simulink model "HVDC_system_original"  (R2024b)
settings: Solver=FixedStepDiscrete  StartTime=0.0  StopTime=1.5  RelTol=1e-4  EnableMultiTasking=on
PreLoadFcn:
  | power_converters_init;
values from neighbouring files (symbols this model uses):
  Clink_3L = Pnom_dc_3L*H_3L*2 /Vnom_dc_3L^2    (= 0.0111111111111)    [HVDC_system_init_original.m]
  fault_distance_km = fault.dist_km    [HVDC_system_init_original.m]
  Fnom = 60    [HVDC_system_init_original.m]
  Ki_Ireg_3L = 15    [HVDC_system_init_original.m]
  Ki_VDCreg_3L = 300    [HVDC_system_init_original.m]
  Kp_Ireg_3L = 0.2/2    (= 0.1)    [HVDC_system_init_original.m]
  Kp_VDCreg_3L = 3    [HVDC_system_init_original.m]
  LimitL_Ireg_3L = -1.5    [HVDC_system_init_original.m]
  LimitL_VDCreg_3L = -1.5    [HVDC_system_init_original.m]
  LimitU_Ireg_3L = 1.5    [HVDC_system_init_original.m]
  LimitU_VDCreg_3L = 1.5    [HVDC_system_init_original.m]
  Lxfo_3L = 0.10    (= 0.1)    [HVDC_system_init_original.m]
  n_g_switch_time = NEVER_TIME    (= 999)    [HVDC_system_init_original.m]
  p_g_switch_time = NEVER_TIME    (= 999)    [HVDC_system_init_original.m]
  p_n_switch_time = NEVER_TIME    (= 999)    [HVDC_system_init_original.m]
  Pnom_3L = Pnom_dc_3L    (= 3000000)    [HVDC_system_init_original.m]
  Pnom_dc_3L = 3e6    (= 3000000)    [HVDC_system_init_original.m]
  Psc_grid = 200e6    (= 200000000)    [HVDC_system_init_original.m]
  R_fault = fault.R    [HVDC_system_init_original.m]
  Rxfo_3L = 0.10/30    (= 0.00333333333333)    [HVDC_system_init_original.m]
  Ts_Control = 50e-6    (= 5e-05)    [HVDC_system_init_original.m]
  Ts_Power = Ts_PWM    (= 5e-06)    [HVDC_system_init_original.m]
  Ts_PWM = 5e-6    (= 5e-06)    [HVDC_system_init_original.m]
  Vnom_dc_3L = 3000    [HVDC_system_init_original.m]
  Vnom_grid = 50e3    (= 50000)    [HVDC_system_init_original.m]
  Vnom_prim_3L = Vnom_grid    (= 50000)    [HVDC_system_init_original.m]
  Vnom_sec_3L = 0.5*Vnom_dc_3L/sqrt(2)*sqrt(3)*m_nom_3L    [HVDC_system_init_original.m]
undefined symbols (not defined in the file or in its folder): D1, Delta, DiscIntNeverNeededParam
libraries: spsSeriesRLCBranchLib x11, powerlib_extras x9, spsVoltageMeasurementLib x8, spsGroundLib x6, spsBreakerLib x4, spsabctodq0Lib x4, spsMeanLib x4, spsPiSectionLineLib x4, spsSecondOrderFilterLib x3, spsThreePhaseVIMeasurementLib x3, spsPLL3phLib x2, spsPWMGenerator3LevelLib x2
(part 1 of 2)
Description:
  | Copyright 2008-2015 The MathWorks, Inc.
settings Model: Creator=MathWorks  LastModifiedBy=ccart030
settings SolverCC: AlgebraicLoopSolver=TrustRegion  AutoInsertRateTranBlk=on
settings DataIOCC: SaveFormat=Array  SaveOutput=off  SignalLogging=off  DSMLogging=off  SaveTime=off  ReturnWorkspaceOutputs=off
settings OptimizationCC: ExpressionDepthLimit=2147483647  LifeSpan=inf
settings DebuggingCC: ConsistencyChecking=warning  UnderspecifiedInitializationDetection=Classic  MergeDetectMultiDrivingBlocksExec=none  TimeAdjustmentMsg=warning  SingleTaskRateTransMsg=warning  VectorMatrixConversionMsg=warning  UnconnectedInputMsg=warning  UnconnectedOutputMsg=warning  UnconnectedLineMsg=warning  AllowSymbolicDim=off  ModelReferenceIOMismatchMessage=warning  StateNameClashWarn=warning  StrictBusMsg=WarnOnBusTreatedAsVector  NonBusSignalsTreatedAsBus=warning  SFUnexpectedBacktrackingDiag=warning  SFNoUnconditionalDefaultTransitionDiag=warning  SFExecutionAtInitializationDiag=none  ArithmeticOperatorsInVariantConditions=warning
settings HardwareCC: ProdBitPerPointer=32  ProdBitPerSizeT=32  ProdBitPerPtrDiffT=32  ProdLargestAtomicFloat=None  ProdIntDivRoundTo=Undefined  ProdEndianess=Unspecified  ProdWordSize=32  ProdHWDeviceType=32-bit Generic
settings ModelReferenceCC: EnableRefExpFcnMdlSchedulingChecks=on  PropagateSignalLabelsOutOfModel=off
settings SFSimCC: SimUseLocalCustomCode=off  CustomCodeUndefinedFunction=UseInterfaceOnly
settings RTWCC: RTWUseLocalCustomCode=off  GPUComputeCapability=3.5
settings CodeAppCC: StateflowObjectComments=on
settings GRTTargetCC: TargetLangStandard=C89/C90 (ANSI)
settings ConfigComp: CovMetricSettings=dw  CovSaveCumulativeToWorkspaceVar=on  CovSaveSingleToWorkspaceVar=on  CovExternalEMLEnable=off  CovSFcnEnable=off
settings SimscapeCC: SimscapeNormalizeSystem=off

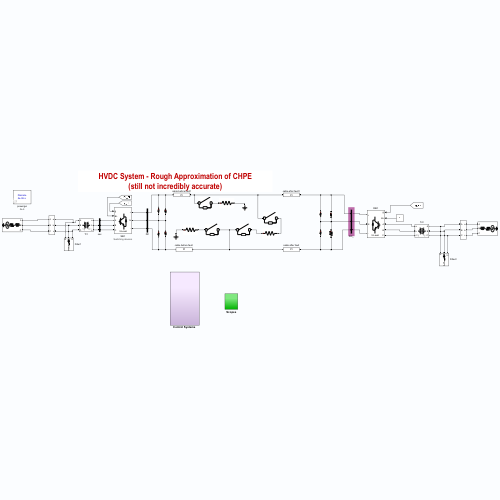
[thumbnail: Simulink's stored preview of the top-level diagram]
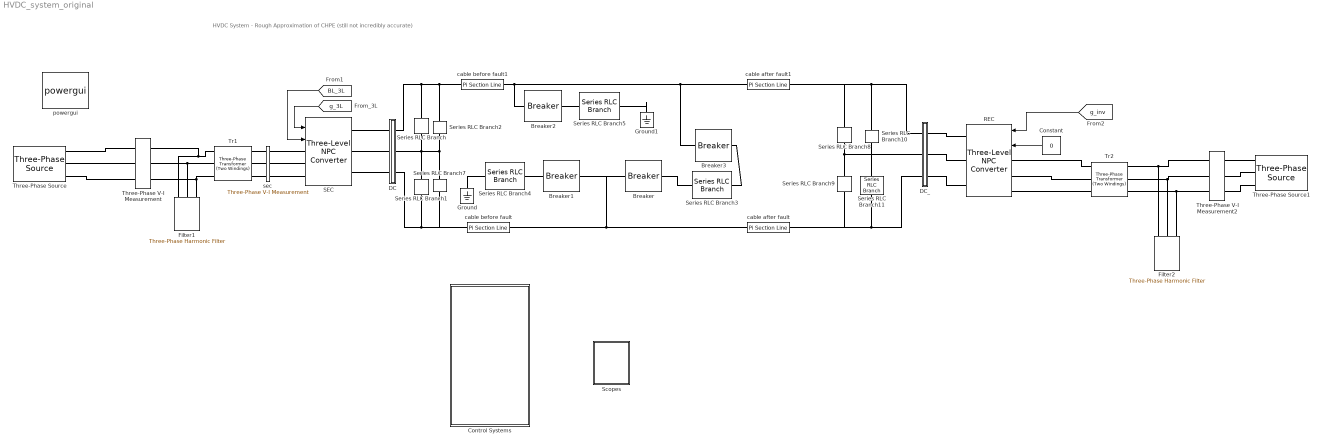
== system HVDC_system_original ==
  note: HVDC System - Rough Approximation of CHPE
      | (still not incredibly accurate)
  Breaker : spsBreakerLib/Breaker  InitialState=0  SwitchingTimes=[p_n_switch_time]  External=off  BreakerResistance=0.01  SnubberResistance=1e6  SnubberCapacitance=inf  Measurements=None  MoreParameters=on  NoBreakLoop=off
  Breaker1 : spsBreakerLib/Breaker  InitialState=0  SwitchingTimes=[n_g_switch_time]  External=off  BreakerResistance=0.01  SnubberResistance=1e6  SnubberCapacitance=inf  Measurements=None  MoreParameters=on  NoBreakLoop=off
  Breaker2 : spsBreakerLib/Breaker  InitialState=0  SwitchingTimes=[p_g_switch_time]  External=off  BreakerResistance=0.01  SnubberResistance=1e6  SnubberCapacitance=inf  Measurements=None  MoreParameters=on  NoBreakLoop=off
  Breaker3 : spsBreakerLib/Breaker  InitialState=0  SwitchingTimes=[p_n_switch_time]  External=off  BreakerResistance=0.01  SnubberResistance=1e6  SnubberCapacitance=inf  Measurements=None  MoreParameters=on  NoBreakLoop=off
  Constant : Constant  Value=0
  "Control Systems " : Subsystem
  DC : Subsystem
  DC_ : Subsystem
  Filter1 : spsThreePhaseHarmonicFilterLib/Three-Phase Harmonic Filter  LConnTagsString=A|B|C  FilterType=Single-tuned  FilterConnection=Y (grounded)  ParNom=[Vnom_prim_3L Fnom]  Qc=Qnom_Filter1  Fr=Fn_Filter1  Frd=[11*60 13*60]  Q=Q_Filter1  Measurements=None
      settings: AttributesFormatString=\n
      settings: LibrarySourceBlock=|
      | sps_lib/Passives/Three-Phase
      | Harmonic Filter
  Filter2 : spsThreePhaseHarmonicFilterLib/Three-Phase Harmonic Filter  LConnTagsString=A|B|C  FilterType=Single-tuned  FilterConnection=Y (grounded)  ParNom=[Vnom_prim_3L Fnom]  Qc=Qnom_Filter1  Fr=Fn_Filter1  Frd=[11*60 13*60]  Q=Q_Filter1  Measurements=None
      settings: AttributesFormatString=\n
      settings: LibrarySourceBlock=|
      | sps_lib/Passives/Three-Phase
      | Harmonic Filter
  Ground : spsGroundLib/Ground  LConnTagsString=a
  Ground1 : spsGroundLib/Ground  LConnTagsString=a
  REC : spsThreeLevelNPCConverterLib/Three-Level NPC Converter  ModelType=Switching devices  Ron=1e-3  Rs=1e6  Cs=inf  Vforward=[0,0]  Ron_Diode=1e-3  Rs_Diode=1e6  Cs_Diode=inf  Vf_Diode=1e-3  Rs_CurrentSource=inf  Ron_ACsource=1e-3
      settings: LibrarySourceBlock=|
      | sps_lib/Power Electronics/Three-Level
      | NPC Converter
  SEC : spsThreeLevelNPCConverterLib/Three-Level NPC Converter  ModelType=Switching devices  Ron=1e-3  Rs=1e6  Cs=inf  Vforward=[ 0, 0 ]  Ron_Diode=1e-3  Rs_Diode=1e6  Cs_Diode=inf  Vf_Diode=1e-3  Rs_CurrentSource=inf  Ron_ACsource=1e-3
      settings: AttributesFormatString=%<ModelType>
      settings: LibrarySourceBlock=|
      | sps_lib/Power Electronics/Three-Level
      | NPC Converter
  Scopes : Subsystem
  Series RLC Branch : spsSeriesRLCBranchLib/Series RLC Branch  LConnTagsString=__new0  RConnTagsString=__new0  BranchType=C  Resistance=1  Inductance=1e-3  SetiL0=off  InitialCurrent=0  Capacitance=Clink_3L  Setx0=on  InitialVoltage=Vc_Initial_3L  Measurements=None
  Series RLC Branch1 : spsSeriesRLCBranchLib/Series RLC Branch  LConnTagsString=__new0  RConnTagsString=__new0  BranchType=C  Resistance=1  Inductance=1e-3  SetiL0=off  InitialCurrent=0  Capacitance=Clink_3L  Setx0=on  InitialVoltage=Vc_Initial_3L  Measurements=None
  Series RLC Branch{2,7,10..11} (4 alike) : spsSeriesRLCBranchLib/Series RLC Branch  LConnTagsString=__new0  RConnTagsString=__new0  BranchType=R  Resistance=Vnom_dc_3L^2/(Pnom_dc_3L*0.01)/2  Inductance=1e-3  SetiL0=off  InitialCurrent=0  Capacitance=1e-6  Setx0=off  InitialVoltage=0  Measurements=None
  Series RLC Branch3 : spsSeriesRLCBranchLib/Series RLC Branch  LConnTagsString=__new0  RConnTagsString=__new0  BranchType=R  Resistance=R_fault  Inductance=1e-3  SetiL0=off  InitialCurrent=0  Capacitance=1e-6  Setx0=off  InitialVoltage=0  Measurements=None
  Series RLC Branch4 : spsSeriesRLCBranchLib/Series RLC Branch  LConnTagsString=__new0  RConnTagsString=__new0  BranchType=R  Resistance=R_fault  Inductance=1e-3  SetiL0=off  InitialCurrent=0  Capacitance=1e-6  Setx0=off  InitialVoltage=0  Measurements=None
  Series RLC Branch5 : spsSeriesRLCBranchLib/Series RLC Branch  LConnTagsString=__new0  RConnTagsString=__new0  BranchType=R  Resistance=R_fault  Inductance=1e-3  SetiL0=off  InitialCurrent=0  Capacitance=1e-6  Setx0=off  InitialVoltage=0  Measurements=None
  Series RLC Branch8 : spsSeriesRLCBranchLib/Series RLC Branch  LConnTagsString=__new0  RConnTagsString=__new0  BranchType=C  Resistance=1  Inductance=1e-3  SetiL0=off  InitialCurrent=0  Capacitance=Clink_3L  Setx0=on  InitialVoltage=Vc_Initial_3L  Measurements=None
  Series RLC Branch9 : spsSeriesRLCBranchLib/Series RLC Branch  LConnTagsString=__new0  RConnTagsString=__new0  BranchType=C  Resistance=1  Inductance=1e-3  SetiL0=off  InitialCurrent=0  Capacitance=Clink_3L  Setx0=off  InitialVoltage=1000  Measurements=None
  Three-Phase V-I Measurement : spsThreePhaseVIMeasurementLib/Three-Phase V-I Measurement  VoltageMeasurement=phase-to-ground  SetLabelV=on  LabelV=Vgrid  Vpu=off  VpuLL=off  CurrentMeasurement=yes  SetLabelI=on  LabelI=Igrid  Ipu=off  Pbase=100e6  Vbase=500e3  OutputType=Complex  PhasorSimulation=off  PSBequivalent=0
  Three-Phase V-I Measurement2 : spsThreePhaseVIMeasurementLib/Three-Phase V-I Measurement  VoltageMeasurement=phase-to-ground  SetLabelV=on  LabelV=Uinv  Vpu=off  VpuLL=off  CurrentMeasurement=yes  SetLabelI=on  LabelI=Iinv  Ipu=off  Pbase=100e6  Vbase=500e3  OutputType=Complex  PhasorSimulation=off  PSBequivalent=0
  Three-Phase Source : spsThreePhaseSourceLib/Three-Phase Source  InternalConnection=Yg  VoltagePhases=off  Voltage=Vnom_grid  PhaseAngle=0  Voltage_phases=[25e3 25e3 25e3]/sqrt(3)  PhaseAngles_phases=[0 -120 +120]  Frequency=Fnom  NonIdealSource=on  SpecifyImpedance=off  Resistance=Vnom_grid*Vnom_grid/Psc_grid/7  Inductance=Vnom_grid*Vnom_grid/Psc_grid/(2*pi*Fnom)  ShortCircuitLevel=100e6  BaseVoltage=Vnom_grid  XRratio=7  BusType=swing  Pref=10e3  Qref=0  Prefabc=[10e3, 10e3, 10e3]  Qrefabc=[0, 0, 0]  Qmin=-inf  Qmax=inf
  Three-Phase Source1 : spsThreePhaseSourceLib/Three-Phase Source  InternalConnection=Yg  VoltagePhases=off  Voltage=Vnom_grid  PhaseAngle=0  Voltage_phases=[25e3 25e3 25e3]/sqrt(3)  PhaseAngles_phases=[0 -120 +120]  Frequency=Fnom  NonIdealSource=on  SpecifyImpedance=off  Resistance=Vnom_grid*Vnom_grid/Psc_grid/7  Inductance=Vnom_grid*Vnom_grid/Psc_grid/(2*pi*Fnom)  ShortCircuitLevel=100e6  BaseVoltage=Vnom_grid  XRratio=7  BusType=swing  Pref=10e3  Qref=0  Prefabc=[10e3, 10e3, 10e3]  Qrefabc=[0, 0, 0]  Qmin=-inf  Qmax=inf
  Tr1 : spsThreePhaseTransformerTwoWindingsLib/Three-Phase Transformer (Two Windings)  Winding1Connection=Yg  Winding2Connection=Delta (D1)  CoreType=Three single-phase transformers  SetSaturation=off  Hysteresis=off  DataFile='hysteresis'  SetInitialFlux=off  Measurements=None  UNITS=pu  NominalPower="[ Pnom_3L,  Fnom ]"  Winding1=[ Vnom_prim_3L ,Rxfo_3L/2 Lxfo_3L/2 ]  Winding2=[ Vnom_sec_3L ,Rxfo_3L/2 Lxfo_3L/2 ]  Rm=Rm_3L  Lm=Lm_3L  L0=0.5  Saturation=[ 0,0 ; 0.0024,1.2 ; 1.0,1.52 ]  InitialFluxes=[ 0.8 , -0.8 , 0.7 ]  BreakLoop=off  DiscreteSolver=Trapezoidal iterative  DataType=off  TransfoNumber=1
  Tr2 : spsThreePhaseTransformerTwoWindingsLib/Three-Phase Transformer (Two Windings)  Winding1Connection=Yg  Winding2Connection=Yg  CoreType=Three single-phase transformers  SetSaturation=off  Hysteresis=off  DataFile='hysteresis'  SetInitialFlux=off  Measurements=None  UNITS=pu  NominalPower="[ Pnom_3L,  Fnom ]"  Winding1=[ Vnom_prim_3L ,Rxfo_3L/2 Lxfo_3L/2 ]  Winding2=[ Vnom_sec_3L ,Rxfo_3L/2 Lxfo_3L/2 ]  Rm=Rm_3L  Lm=Lm_3L  L0=0.5  Saturation=[ 0,0 ; 0.0024,1.2 ; 1.0,1.52 ]  InitialFluxes=[ 0.8 , -0.8 , 0.7 ]  BreakLoop=off  DiscreteSolver=Trapezoidal iterative  DataType=off  TransfoNumber=1
  cable after fault : spsPiSectionLineLib/Pi Section Line  LConnTagsString=__new0  RConnTagsString=__new0  Phases=1  PiSections=2  Length=546-fault_distance_km  Frequency=Fnom  Resistance=1.3900e-004  Inductance=1.5900e-005  Capacitance=2.3100e-005  SpecifyConductance=off  Conductance=0  Measurements=None  Measurements2=None
      settings: LibrarySourceBlock=sps_lib/Power Grid Elements/Pi Section Line
  cable after fault1 : spsPiSectionLineLib/Pi Section Line  LConnTagsString=__new0  RConnTagsString=__new0  Phases=1  PiSections=2  Length=546-fault_distance_km  Frequency=Fnom  Resistance=1.3900e-004  Inductance=1.5900e-005  Capacitance=2.3100e-005  SpecifyConductance=off  Conductance=0  Measurements=None  Measurements2=None
      settings: LibrarySourceBlock=sps_lib/Power Grid Elements/Pi Section Line
  "cable before fault " : spsPiSectionLineLib/Pi Section Line  LConnTagsString=__new0  RConnTagsString=__new0  Phases=1  PiSections=2  Length=fault_distance_km  Frequency=Fnom  Resistance=1.3900e-004  Inductance=1.5900e-005  Capacitance=2.3100e-005  SpecifyConductance=off  Conductance=0  Measurements=None  Measurements2=None
      settings: LibrarySourceBlock=sps_lib/Power Grid Elements/Pi Section Line
  cable before fault1 : spsPiSectionLineLib/Pi Section Line  LConnTagsString=__new0  RConnTagsString=__new0  Phases=1  PiSections=2  Length=fault_distance_km  Frequency=Fnom  Resistance=1.3900e-004  Inductance=1.5900e-005  Capacitance=2.3100e-005  SpecifyConductance=off  Conductance=0  Measurements=None  Measurements2=None
      settings: LibrarySourceBlock=sps_lib/Power Grid Elements/Pi Section Line
  powergui : sps_lib/powergui  Priority=1  SimulationMode=Discrete  SampleTime=5e-6  frequency=60  Iterations=50  frequencyindice=60  Pbase=100e6  ErrMax=1e-4  UnitsV=kV  UnitsW=MW  buscounter=0  FunctionMessages=off  echomessages=off  EnableUseOfTLC=off  CurrentSourceSwitches=off  DisableSnubberDevices=off  DisableRonSwitches=off  DisableVfSwitches=off  DisplayEquations=off  AutomaticDiscreteSolvers=off  SolverType=Tustin/Backward Euler (TBE)  Interpol=off  ExternalGateDelay=off  methode=on  Ts=100  x0status=steady  SPID=off  SwTol=0  HookPort=off  NonlinearTolerance=1e-4  nMaxIteration=100  ContinueOnMaxIteration=off  RestoreLinks=warning  ResistiveCurrentMeasurement=off  Frange=[0:2:500]  Ylog=off  Xlog=on  ShowGrid=off  save=off  variable=ZData  structure=VIPFB  ZoomFFT=on  StartTime=0.87  cycles=1  DisplayStyle=1  fundamental=50  FreqAxis=on  MaxFrequency=5000  frequencyindicesteady=1  RmsSteady=2  display=off
      settings: AttributesFormatString=%<SampleTime>
  sec : spsThreePhaseVIMeasurementLib/Three-Phase V-I Measurement  VoltageMeasurement=phase-to-phase  SetLabelV=on  LabelV=Vsec_3L_LL  Vpu=off  VpuLL=off  CurrentMeasurement=no  SetLabelI=on  LabelI=Isec  Ipu=off  Pbase=100e6  Vbase=500e3  OutputType=Complex  PhasorSimulation=off  PSBequivalent=0
  wires:
  [g_3L] -> SEC/1
  [BL_3L] -> SEC/2
  Constant/1 -> REC/2
  [g_inv] -> REC/1
  connections:
  Filter1/LConn1 -- Three-Phase V-I Measurement/RConn1 -- Tr1/LConn1
  Filter1/LConn3 -- Three-Phase V-I Measurement/RConn3 -- Tr1/LConn3
  sec/RConn1 -- Tr1/RConn1
  Tr1/RConn2 -- sec/RConn2
  Tr1/RConn3 -- sec/RConn3
  SEC/LConn1 -- sec/LConn1
  SEC/LConn2 -- sec/LConn2
  SEC/LConn3 -- sec/LConn3
  Three-Phase Source/RConn1 -- Three-Phase V-I Measurement/LConn1
  Three-Phase Source/RConn2 -- Three-Phase V-I Measurement/LConn2
  Three-Phase Source/RConn3 -- Three-Phase V-I Measurement/LConn3
  SEC/RConn1 -- DC/LConn1
  SEC/RConn2 -- DC/LConn2
  SEC/RConn3 -- DC/LConn3
  Series RLC Branch1/RConn1 -- Series RLC Branch7/RConn1 -- "cable before fault "/LConn1 -- DC/RConn3
  Series RLC Branch1/LConn1 -- DC/RConn2 -- Series RLC Branch7/LConn1 -- Series RLC Branch2/RConn1 -- Series RLC Branch/RConn1
  Filter1/LConn2 -- Three-Phase V-I Measurement/RConn2 -- Tr1/LConn2
  Tr2/RConn1 -- REC/LConn1
  REC/LConn2 -- Tr2/RConn2
  REC/LConn3 -- Tr2/RConn3
  DC_/RConn1 -- REC/RConn1
  DC_/RConn2 -- REC/RConn2
  DC_/RConn3 -- REC/RConn3
  Series RLC Branch8/RConn1 -- Series RLC Branch11/LConn1 -- DC_/LConn2 -- Series RLC Branch10/RConn1 -- Series RLC Branch9/LConn1
  Series RLC Branch2/LConn1 -- cable before fault1/LConn1 -- DC/RConn1 -- Series RLC Branch/LConn1
  Three-Phase V-I Measurement2/LConn2 -- Filter2/LConn2 -- Tr2/LConn2
  Three-Phase V-I Measurement2/LConn1 -- Tr2/LConn1 -- Filter2/LConn1
  Three-Phase V-I Measurement2/LConn3 -- Filter2/LConn3 -- Tr2/LConn3
  Three-Phase Source1/RConn1 -- Three-Phase V-I Measurement2/RConn1
  Three-Phase Source1/RConn2 -- Three-Phase V-I Measurement2/RConn2
  Three-Phase Source1/RConn3 -- Three-Phase V-I Measurement2/RConn3
  Series RLC Branch10/LConn1 -- cable after fault1/RConn1 -- Series RLC Branch8/LConn1 -- DC_/LConn1
  Series RLC Branch11/RConn1 -- Series RLC Branch9/RConn1 -- cable after fault/RConn1 -- DC_/LConn3
  "cable before fault "/RConn1 -- Breaker/LConn1 -- Breaker1/RConn1 -- cable after fault/LConn1
  cable before fault1/RConn1 -- Breaker3/LConn1 -- cable after fault1/LConn1 -- Breaker2/LConn1
  Breaker/RConn1 -- Series RLC Branch3/LConn1
  Series RLC Branch4/RConn1 -- Breaker1/LConn1
  Series RLC Branch3/RConn1 -- Breaker3/RConn1
  Ground/LConn1 -- Series RLC Branch4/LConn1
  Series RLC Branch5/LConn1 -- Breaker2/RConn1
  Ground1/LConn1 -- Series RLC Branch5/RConn1

== system HVDC_system_original/Control Systems  ==
  REC Control : Subsystem
  SEC Control : Subsystem

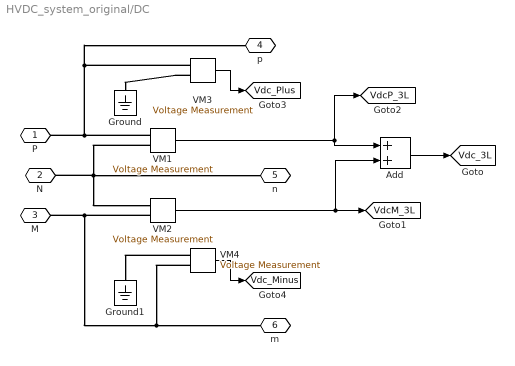
== system HVDC_system_original/DC ==
  Add : Sum
  Ground : spsGroundLib/Ground  LConnTagsString=a
  Ground1 : spsGroundLib/Ground  LConnTagsString=a
  VM{1..4} (4 alike) : spsVoltageMeasurementLib/Voltage Measurement  PhasorSimulation=off  OutputType=Complex  PSBequivalent=0
  P : PMIOPort  Side=Left
  N : PMIOPort  Port=2  Side=Left
  M : PMIOPort  Port=3  Side=Left
  p : PMIOPort  Port=4  Side=Right
  n : PMIOPort  Port=5  Side=Right
  m : PMIOPort  Port=6  Side=Right
  tag scope: VdcM_3L=global, VdcP_3L=global, Vdc_3L=global, Vdc_Minus=global, Vdc_Plus=global
  wires:
  VM1/1 -> [VdcP_3L], Add/1
  VM2/1 -> Add/2, [VdcM_3L]
  Add/1 -> [Vdc_3L]
  VM3/1 -> [Vdc_Plus]
  VM4/1 -> [Vdc_Minus]
  connections:
  VM1/LConn1 -- VM3/LConn1 -- p/RConn1 -- P/RConn1
  VM2/LConn2 -- VM4/LConn2 -- m/RConn1 -- M/RConn1
  VM1/LConn2 -- n/RConn1 -- VM2/LConn1 -- N/RConn1
  VM3/LConn2 -- Ground/LConn1
  VM4/LConn1 -- Ground1/LConn1

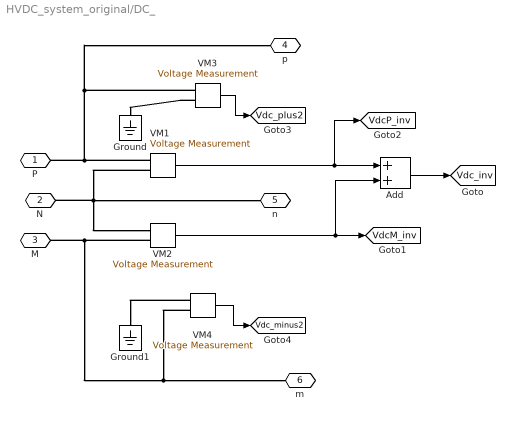
== system HVDC_system_original/DC_ ==
  Add : Sum
  Ground : spsGroundLib/Ground  LConnTagsString=a
  Ground1 : spsGroundLib/Ground  LConnTagsString=a
  VM{1..4} (4 alike) : spsVoltageMeasurementLib/Voltage Measurement  PhasorSimulation=off  OutputType=Complex  PSBequivalent=0
  P : PMIOPort  Side=Left
  N : PMIOPort  Port=2  Side=Left
  M : PMIOPort  Port=3  Side=Left
  p : PMIOPort  Port=4  Side=Right
  n : PMIOPort  Port=5  Side=Right
  m : PMIOPort  Port=6  Side=Right
  tag scope: VdcM_inv=global, VdcP_inv=global, Vdc_inv=global, Vdc_minus2=global, Vdc_plus2=global
  wires:
  VM1/1 -> [VdcP_inv], Add/1
  VM2/1 -> Add/2, [VdcM_inv]
  Add/1 -> [Vdc_inv]
  VM3/1 -> [Vdc_plus2]
  VM4/1 -> [Vdc_minus2]
  connections:
  VM1/LConn1 -- VM3/LConn1 -- p/RConn1 -- P/RConn1
  VM2/LConn2 -- VM4/LConn2 -- m/RConn1 -- M/RConn1
  VM1/LConn2 -- n/RConn1 -- VM2/LConn1 -- N/RConn1
  VM3/LConn2 -- Ground/LConn1
  VM4/LConn1 -- Ground1/LConn1

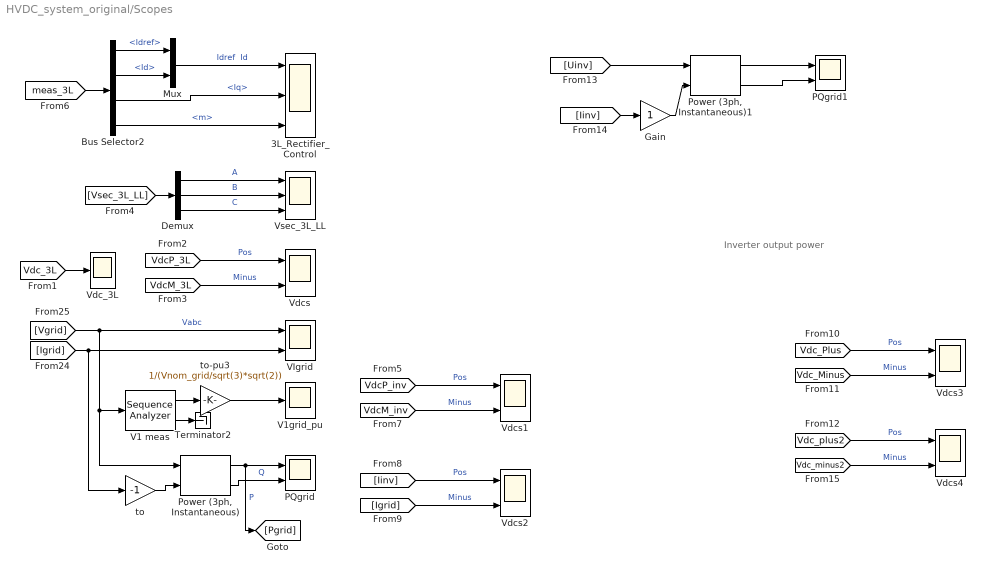
== system HVDC_system_original/Scopes ==
  note: Inverter output power
  3L_Rectifier_Control : Scope  NumInputPorts=3
  Bus Selector2 : BusSelector  OutputSignals=Idref,Id,Iq,m
  Demux : Demux  Outputs=3
  Gain : Gain
  Mux : Mux  Inputs=2
  PQgrid : Scope  NumInputPorts=2
  PQgrid1 : Scope  NumInputPorts=2
  "Power (3ph, Instantaneous)" : spsPower3phInstantaneousLib/Power (3ph, Instantaneous)
  "Power (3ph, Instantaneous)1" : spsPower3phInstantaneousLib/Power (3ph, Instantaneous)
  Terminator2 : Terminator
  V1 meas : spsSequenceAnalyzerLib/Sequence Analyzer  Freq=Fnom  n=1  seq=Positive  InInit=[1, 0]  Ts=Ts_Power
      settings: LibrarySourceBlock=sps_lib/Sensors and Measurements/Sequence Analyzer
  V1grid_pu : Scope
  VIgrid : Scope  NumInputPorts=2
  Vdc_3L : Scope
  Vdcs{,1..4} (5 alike) : Scope  NumInputPorts=2
  Vsec_3L_LL : Scope  NumInputPorts=3
  to : Gain  Gain=-1
  to-pu3 : Gain  Gain=1/(Vnom_grid/sqrt(3)*sqrt(2))
  wires:
  [meas_3L] -> Bus Selector2/1
  "Power (3ph, Instantaneous)"/1 -> [Pgrid], PQgrid/1  "P"
  V1 meas/2 -> Terminator2/1
  V1 meas/1 -> to-pu3/1
  to-pu3/1 -> V1grid_pu/1
  Mux/1 -> 3L_Rectifier_Control/1  "Idref  Id"
  Bus Selector2/1 -> Mux/1  "<Idref>"
  Bus Selector2/2 -> Mux/2  "<Id>"
  Bus Selector2/4 -> 3L_Rectifier_Control/3  "<m>"
  Bus Selector2/3 -> 3L_Rectifier_Control/2  "<Iq>"
  [Vdc_3L] -> Vdc_3L/1
  [VdcP_3L] -> Vdcs/1  "Pos"
  [VdcM_3L] -> Vdcs/2  "Minus"
  [Vsec_3L_LL] -> Demux/1
  Demux/1 -> Vsec_3L_LL/1  "A"
  Demux/2 -> Vsec_3L_LL/2  "B"
  Demux/3 -> Vsec_3L_LL/3  "C"
  "Power (3ph, Instantaneous)"/2 -> PQgrid/2  "Q"
  [Igrid] -> VIgrid/2, to/1
  [Vgrid] -> VIgrid/1, "Power (3ph, Instantaneous)"/1, V1 meas/1  "Vabc"
  [Uinv] -> "Power (3ph, Instantaneous)1"/1
  [Iinv] -> Gain/1
  to/1 -> "Power (3ph, Instantaneous)"/2
  Gain/1 -> "Power (3ph, Instantaneous)1"/2
  "Power (3ph, Instantaneous)1"/1 -> PQgrid1/1
  "Power (3ph, Instantaneous)1"/2 -> PQgrid1/2
  [VdcM_inv] -> Vdcs1/2  "Minus"
  [VdcP_inv] -> Vdcs1/1  "Pos"
  [Igrid] -> Vdcs2/2  "Minus"
  [Iinv] -> Vdcs2/1  "Pos"
  [Vdc_Minus] -> Vdcs3/2  "Minus"
  [Vdc_Plus] -> Vdcs3/1  "Pos"
  [Vdc_plus2] -> Vdcs4/1  "Pos"
  [Vdc_minus2] -> Vdcs4/2  "Minus"

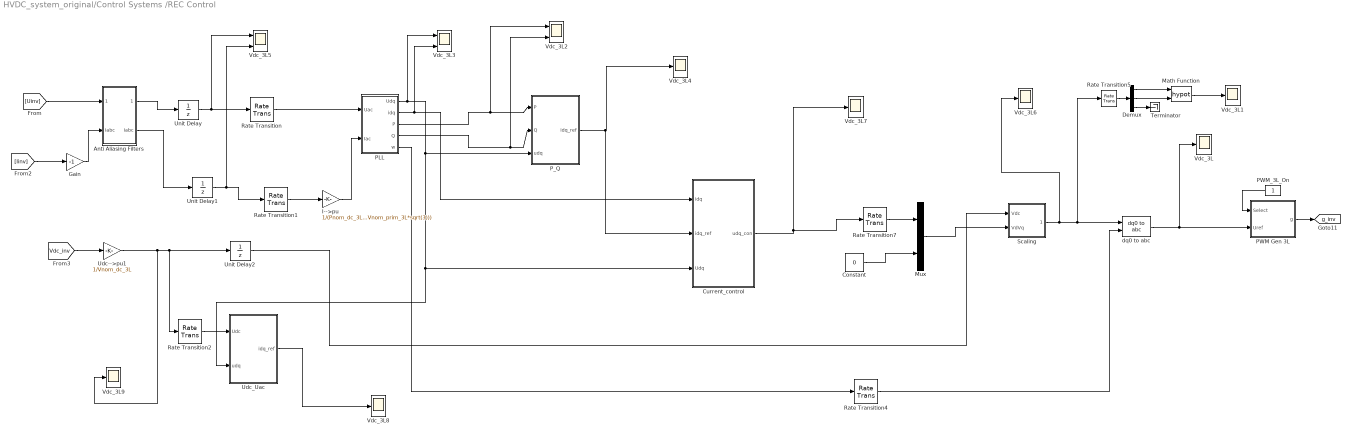
== system HVDC_system_original/Control Systems /REC Control ==
  Anti Aliasing Filters : Subsystem  mask(Anti-aliasing (2nd order lowpass)){Fc=800, Ts=Ts_Power}
      mask prompts: Fc "Cut-off frequency (Hz):"; Ts "Sample time:"
  Constant : Constant  Value=0  SampleTime=Ts_PWM
  Current_control : Subsystem
  Demux : Demux  Outputs=3
  Gain : Gain  Gain=-1
  I-->pu : Gain  Gain=1/(Pnom_dc_3L*sqrt(2)/(Vnom_prim_3L*sqrt(3)))
  Math Function : Math  Operator=hypot  SignedPower=on
  Mux : Mux  Inputs=2
  PLL : Subsystem
  PWM Gen 3L : Subsystem
  PWM_3L_On : Constant
      settings: AttributesFormatString=%<Tag>
  P_Q : Subsystem
  Rate Transition{,1..2,5} (4 alike) : RateTransition  OutPortSampleTime=Ts_Control
  Rate Transition4 : RateTransition  OutPortSampleTime=Ts_PWM
  Rate Transition7 : RateTransition  OutPortSampleTime=Ts_PWM
  Scaling : Subsystem
  Terminator : Terminator
  Udc-->pu1 : Gain  Gain=1/Vnom_dc_3L
  Udc_Uac : Subsystem
  Unit Delay : UnitDelay  SampleTime=Ts_Power  HasFrameUpgradeWarning=on
  Unit Delay1 : UnitDelay  SampleTime=Ts_Power  HasFrameUpgradeWarning=on
  Unit Delay2 : UnitDelay  SampleTime=Ts_PWM  HasFrameUpgradeWarning=on
  Vdc_3L{,1,4,6..9} (7 alike) : Scope
  Vdc_3L2 : Scope  NumInputPorts=2
  Vdc_3L3 : Scope  NumInputPorts=2
  Vdc_3L5 : Scope  NumInputPorts=2
  dq0 to abc : spsdq0toabcLib/dq0 to abc  Alignment=90 degrees behind phase A axis
  tag scope: g_inv=global
  wires:
  [Vdc_inv] -> Udc-->pu1/1
  Anti Aliasing Filters/2(Iabc) -> Unit Delay1/1
  Rate Transition1/1 -> I-->pu/1
  Unit Delay/1 -> Vdc_3L5/1, Rate Transition/1
  Rate Transition/1 -> PLL/1(Uac)
  Unit Delay1/1 -> Vdc_3L5/2, Rate Transition1/1
  I-->pu/1 -> PLL/2(Iac)
  PLL/3(P) -> P_Q/1(P), Vdc_3L2/1
  PLL/4(Q) -> Vdc_3L2/2, P_Q/2(Q)
  PLL/2(idq) -> Vdc_3L3/2, Current_control/1(idq)
  P_Q/1(idq_ref) -> Current_control/2(idq_ref), Vdc_3L4/1
  PLL/1(Udq) -> Vdc_3L3/1, P_Q/3(udq), Current_control/3(Udq), Udc_Uac/2(udq)
  Current_control/1(udq_con) -> Vdc_3L7/1, Rate Transition7/1
  Constant/1 -> Mux/2
  PWM Gen 3L/1(g) -> [g_inv]
  PWM_3L_On/1 -> PWM Gen 3L/1(Select)
  dq0 to abc/1 -> Vdc_3L/1, PWM Gen 3L/2(Uref)
  Scaling/1(VdVq*) -> Vdc_3L6/1, Rate Transition5/1, dq0 to abc/1
  Demux/3 -> Terminator/1
  Demux/2 -> Math Function/2
  Demux/1 -> Math Function/1
  Rate Transition5/1 -> Demux/1
  Math Function/1 -> Vdc_3L1/1
  PLL/5(w) -> Rate Transition4/1
  Mux/1 -> Scaling/2(VdVq)
  Rate Transition4/1 -> dq0 to abc/2
  Unit Delay2/1 -> Scaling/1(Vdc)
  Rate Transition7/1 -> Mux/1
  [Uinv] -> Anti Aliasing Filters/1(Vabc)
  Anti Aliasing Filters/1(" Vabc") -> Unit Delay/1
  [Iinv] -> Gain/1
  Gain/1 -> Anti Aliasing Filters/2("Iabc ")
  Udc-->pu1/1 -> Vdc_3L9/1, Unit Delay2/1, Rate Transition2/1
  Rate Transition2/1 -> Udc_Uac/1(Udc)
  Udc_Uac/1(idq_ref) -> Vdc_3L8/1

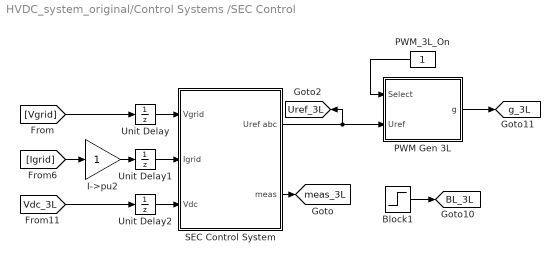
== system HVDC_system_original/Control Systems /SEC Control ==
  Block1 : Step  Time=999  SampleTime=Ts_Power
  I->pu2 : Gain  SaturateOnIntegerOverflow=on  OutDataTypeStr=Inherit: Same as input  ParamDataTypeStr=Inherit: Same as input
  PWM Gen 3L : Subsystem
  PWM_3L_On : Constant
      settings: AttributesFormatString=%<Tag>
  SEC Control System : Subsystem
  Unit Delay : UnitDelay  SampleTime=Ts_Power  HasFrameUpgradeWarning=on
  Unit Delay1 : UnitDelay  SampleTime=Ts_Power  HasFrameUpgradeWarning=on
  Unit Delay2 : UnitDelay  SampleTime=Ts_Power  HasFrameUpgradeWarning=on
  tag scope: BL_3L=global, Uref_3L=global, g_3L=global, meas_3L=global
  wires:
  SEC Control System/2(meas) -> [meas_3L]
  Block1/1 -> [BL_3L]
  [Vgrid] -> Unit Delay/1
  SEC Control System/1(Uref abc) -> [Uref_3L], PWM Gen 3L/2(Uref)
  [Vdc_3L] -> Unit Delay2/1
  Unit Delay1/1 -> SEC Control System/2(Igrid)
  Unit Delay2/1 -> SEC Control System/3(Vdc)
  Unit Delay/1 -> SEC Control System/1(Vgrid)
  PWM Gen 3L/1(g) -> [g_3L]
  PWM_3L_On/1 -> PWM Gen 3L/1(Select)
  I->pu2/1 -> Unit Delay1/1
  [Igrid] -> I->pu2/1

== system HVDC_system_original/Control Systems /REC Control/Anti Aliasing Filters ==
  Vabc : Inport  PortDimensions=3
  "Iabc " : Inport  Port=2  PortDimensions=3
  2nd-Order Filter : powerlib_extras/Discrete  Control Blocks/Discrete  2nd-Order Filter  FilterType=Lowpass  Fo=Fc  Zeta=0.707  Ts=Ts  Initialize=off  Vac_Init=[0.8 -25 60]  Vdc_Init=-0.4  PlotResponse=off  param1=[1 120 0.1]
  2nd-Order Filter{1..5} (5 alike) : powerlib_extras/Discrete  Control Blocks/Discrete  2nd-Order Filter  FilterType=Lowpass  Fo=Fc  Zeta=0.707  Ts=Ts  Initialize=off  Vac_Init=[0.8 -25 60]  Vdc_Init=-0.4  PlotResponse=off  param1=[1 5000 0.1]
  Demux : Demux  Outputs=3
      settings: DisplayOption=none
  Demux1 : Demux  Outputs=3
      settings: DisplayOption=none
  Mux : Mux  Inputs=3
  Mux1 : Mux  Inputs=3
  " Vabc" : Outport
  Iabc : Outport  Port=2
  wires:
  "Iabc "/1 -> Demux1/1
  Demux1/2 -> 2nd-Order Filter4/1
  Demux1/3 -> 2nd-Order Filter5/1
  2nd-Order Filter5/1 -> Mux1/3
  2nd-Order Filter4/1 -> Mux1/2
  Mux1/1 -> Iabc/1
  2nd-Order Filter3/1 -> Mux1/1
  Demux1/1 -> 2nd-Order Filter3/1
  Demux/2 -> 2nd-Order Filter1/1
  Demux/3 -> 2nd-Order Filter2/1
  2nd-Order Filter2/1 -> Mux/3
  2nd-Order Filter1/1 -> Mux/2
  Mux/1 -> " Vabc"/1
  2nd-Order Filter/1 -> Mux/1
  Vabc/1 -> Demux/1
  Demux/1 -> 2nd-Order Filter/1

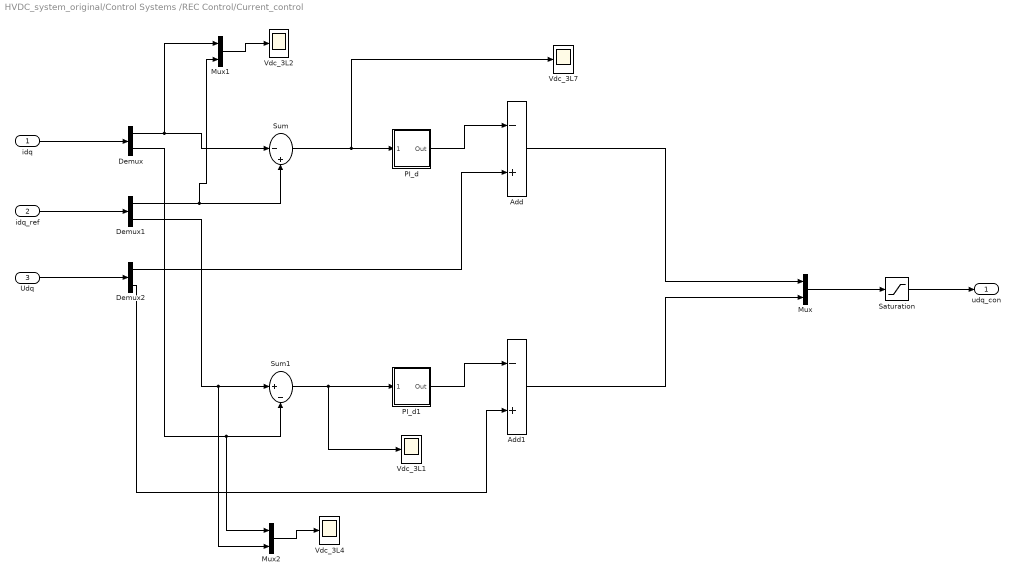
== system HVDC_system_original/Control Systems /REC Control/Current_control ==
  idq : Inport
  idq_ref : Inport  Port=2
  Udq : Inport  Port=3
  Add : Sum  Inputs=-+
  Add1 : Sum  Inputs=-+
  Demux : Demux  Outputs=2
  Demux1 : Demux  Outputs=2
  Demux2 : Demux  Outputs=2
  Mux : Mux  Inputs=2
  Mux1 : Mux  Inputs=2
  Mux2 : Mux  Inputs=2
  PI_d : Subsystem  DialogController=POWERSYS.PowerSysDialog  mask(Discrete PI Controller){Kp=Kp_Ireg_3L, Ki=Ki_Ireg_3L, Par_Limits=[ LimitU_Ireg_3L LimitL_Ireg_3L ], Init=0.5, Ts=Ts_Control}
      mask prompts: Kp "Proportional gain (Kp):"; Ki "Integral gain (Ki):"; Par_Limits "Output limits: [ Upper   Lower ]"; Init "Output initial value:"; Ts "Sample time:"
      mask help: This block implements a discrete PI controller.
      mask init:
      | UpperLimit=Par_Limits(1);
      | LowerLimit=Par_Limits(2);
      mask Display: disp('PI');
  PI_d1 : Subsystem  DialogController=POWERSYS.PowerSysDialog  mask(Discrete PI Controller){Kp=Kp_Ireg_3L, Ki=Ki_Ireg_3L, Par_Limits=[ LimitU_Ireg_3L LimitL_Ireg_3L ], Init=0.12, Ts=Ts_Control}
      mask prompts: Kp "Proportional gain (Kp):"; Ki "Integral gain (Ki):"; Par_Limits "Output limits: [ Upper   Lower ]"; Init "Output initial value:"; Ts "Sample time:"
      mask help: This block implements a discrete PI controller.
      mask init:
      | UpperLimit=Par_Limits(1);
      | LowerLimit=Par_Limits(2);
      mask Display: disp('PI');
  Saturation : Saturate  UpperLimit=LimitU_Ireg_3L  LowerLimit=LimitL_Ireg_3L
  Sum : Sum  Inputs=|-+
  Sum1 : Sum  Inputs=|+-
  Vdc_3L{1..2,4,7} (4 alike) : Scope
  udq_con : Outport
  wires:
  idq/1 -> Demux/1
  idq_ref/1 -> Demux1/1
  Udq/1 -> Demux2/1
  Demux1/1 -> Mux1/2, Sum/2
  Demux/1 -> Mux1/1, Sum/1
  Sum/1 -> Vdc_3L7/1, PI_d/1(Error)
  PI_d/1(Out) -> Add/1
  Demux2/1 -> Add/2
  Sum1/1 -> Vdc_3L1/1, PI_d1/1(Error)
  PI_d1/1(Out) -> Add1/1
  Demux2/2 -> Add1/2
  Demux1/2 -> Mux2/2, Sum1/1
  Mux/1 -> Saturation/1
  Add/1 -> Mux/1
  Add1/1 -> Mux/2
  Saturation/1 -> udq_con/1
  Mux1/1 -> Vdc_3L2/1
  Demux/2 -> Mux2/1, Sum1/2
  Mux2/1 -> Vdc_3L4/1

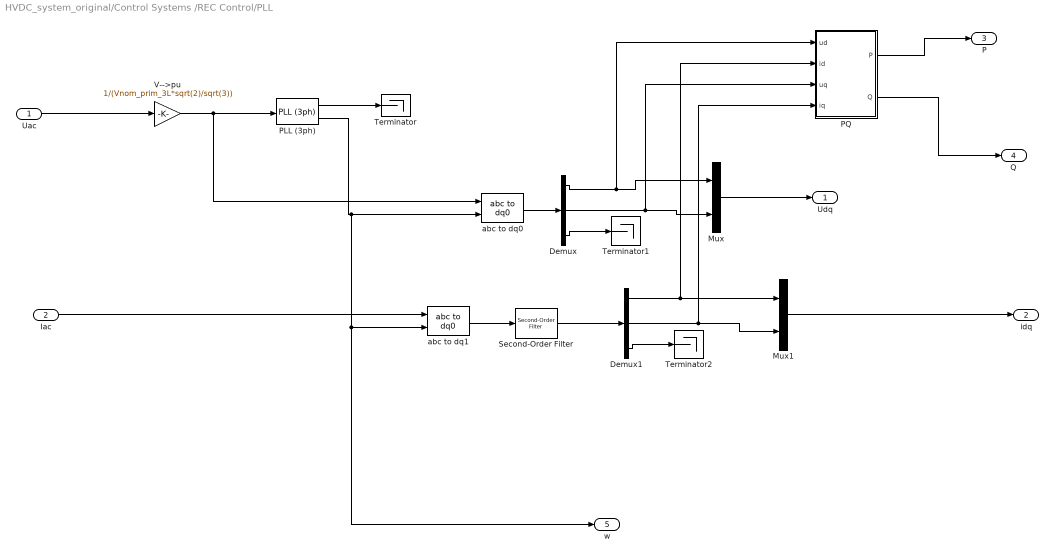
== system HVDC_system_original/Control Systems /REC Control/PLL ==
  Uac : Inport
  Iac : Inport  Port=2
  Demux : Demux  Outputs=3
  Demux1 : Demux  Outputs=3
  Mux : Mux  Inputs=2
  Mux1 : Mux  Inputs=2
  PLL (3ph) : spsPLL3phLib/PLL (3ph)  Fmin=45  Par_Init=[0, Fnom]  ParK=[180, 3200, 1]  TcD=1e-4  MaxRateChangeFreq=12  FilterCutOffFreq=25  Ts=Ts_Control  AGC=on
  PQ : Subsystem
  Second-Order Filter : spsSecondOrderFilterLib/Second-Order Filter  FilterType=Lowpass  Fo=Freq_Filter  Zeta=1  Ts=Ts_Control  Initialize=off  Vac_Init="[0,  0,  60]"  Vdc_Init=0  PlotResponse=off  FreqRange=[0, 500, 1]
      settings: LibrarySourceBlock=|
      | sps_lib/Control/Filters/Second-Order
      | Filter
  Terminator : Terminator
  Terminator1 : Terminator
  Terminator2 : Terminator
  V-->pu : Gain  Gain=1/(Vnom_prim_3L*sqrt(2)/sqrt(3))
  abc to dq0 : spsabctodq0Lib/abc to dq0  Alignment=90 degrees behind phase A axis
  abc to dq1 : spsabctodq0Lib/abc to dq0  Alignment=90 degrees behind phase A axis
  Udq : Outport
  idq : Outport  Port=2
  P : Outport  Port=3
  Q : Outport  Port=4
  w : Outport  Port=5
  wires:
  Uac/1 -> V-->pu/1
  V-->pu/1 -> abc to dq0/1, PLL (3ph)/1
  PLL (3ph)/1 -> Terminator/1
  PLL (3ph)/2 -> abc to dq1/2, w/1, abc to dq0/2
  abc to dq0/1 -> Demux/1
  Demux/3 -> Terminator1/1
  Demux/1 -> PQ/1(ud), Mux/1
  Demux/2 -> PQ/3(uq), Mux/2
  Iac/1 -> abc to dq1/1
  abc to dq1/1 -> Second-Order Filter/1
  Demux1/3 -> Terminator2/1
  Demux1/1 -> PQ/2(id), Mux1/1
  Demux1/2 -> Mux1/2, PQ/4(iq)
  Mux/1 -> Udq/1
  Mux1/1 -> idq/1
  PQ/2(Q) -> Q/1
  PQ/1(P) -> P/1
  Second-Order Filter/1 -> Demux1/1

== system HVDC_system_original/Control Systems /REC Control/PWM Gen 3L ==
  Select : Inport
  Uref : Inport  Port=2
  PWMgen - Averaging : Subsystem
  Pavg_3L : Subsystem
  Switch : Switch  Threshold=1.5  SaturateOnIntegerOverflow=off  InputSameDT=off
  g : Outport
  wires:
  Select/1 -> PWMgen - Averaging/Enable, Switch/2
  PWMgen - Averaging/1(g1_avg) -> Pavg_3L/1(g1)
  Switch/1 -> g/1
  PWMgen - Averaging/2(g4_avg) -> Pavg_3L/2(g4)
  PWMgen - Averaging/3(P) -> Switch/3
  Uref/1 -> PWMgen - Averaging/1(Uref)
  Pavg_3L/1(g) -> Switch/1

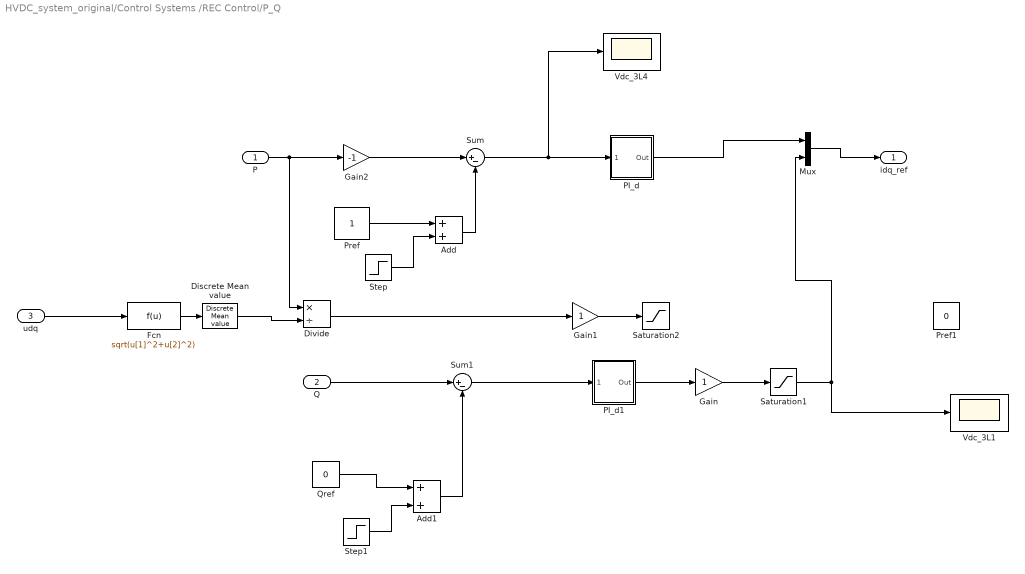
== system HVDC_system_original/Control Systems /REC Control/P_Q ==
  P : Inport
  Q : Inport  Port=2
  udq : Inport  Port=3
  Add : Sum
  Add1 : Sum
  Discrete Mean value : powerlib_extras/Discrete Measurements/Discrete  Mean value  Freq=Fnom  Vinit=1  Ts=Ts_Control
  Divide : Product  Inputs=*/
  Fcn : Fcn  Expr=sqrt(u[1]^2+u[2]^2)  SampleTime=Ts_Control
  Gain : Gain
  Gain1 : Gain
  Gain2 : Gain  Gain=-1
  Mux : Mux  Inputs=2
  PI_d : Subsystem  DialogController=POWERSYS.PowerSysDialog  mask(Discrete PI Controller){Kp=0.3, Ki=40, Par_Limits=[1.15 -1.15], Init=-1, Ts=Ts_Control}
      mask prompts: Kp "Proportional gain (Kp):"; Ki "Integral gain (Ki):"; Par_Limits "Output limits: [ Upper   Lower ]"; Init "Output initial value:"; Ts "Sample time:"
      mask help: This block implements a discrete PI controller.
      mask init:
      | UpperLimit=Par_Limits(1);
      | LowerLimit=Par_Limits(2);
      mask Display: disp('PI');
  PI_d1 : Subsystem  DialogController=POWERSYS.PowerSysDialog  mask(Discrete PI Controller){Kp=0.4, Ki=30, Par_Limits=[1 -1], Init=0, Ts=Ts_Control}
      mask prompts: Kp "Proportional gain (Kp):"; Ki "Integral gain (Ki):"; Par_Limits "Output limits: [ Upper   Lower ]"; Init "Output initial value:"; Ts "Sample time:"
      mask help: This block implements a discrete PI controller.
      mask init:
      | UpperLimit=Par_Limits(1);
      | LowerLimit=Par_Limits(2);
      mask Display: disp('PI');
  Pref : Constant
  Pref1 : Constant  Value=0
  Qref : Constant  Value=0
  Saturation1 : Saturate  UpperLimit=1  LowerLimit=-1
  Saturation2 : Saturate  UpperLimit=1  LowerLimit=-1
  Step : Step  After=-0.2  SampleTime=Ts_Control
  Step1 : Step  Time=1.2  After=0.2  SampleTime=Ts_Control
  Sum : Sum  Inputs=|+-
  Sum1 : Sum  Inputs=|+-
  Vdc_3L1 : Scope
  Vdc_3L4 : Scope
  idq_ref : Outport
  wires:
  Sum/1 -> Vdc_3L4/1, PI_d/1(Error)
  PI_d1/1(Out) -> Gain/1
  Q/1 -> Sum1/1
  Sum1/1 -> PI_d1/1(Error)
  Mux/1 -> idq_ref/1
  Gain/1 -> Saturation1/1
  Fcn/1 -> Discrete Mean value/1
  udq/1 -> Fcn/1
  P/1 -> Gain2/1, Divide/1
  Discrete Mean value/1 -> Divide/2
  Divide/1 -> Gain1/1
  Gain1/1 -> Saturation2/1
  Saturation1/1 -> Mux/2, Vdc_3L1/1
  PI_d/1(Out) -> Mux/1
  Gain2/1 -> Sum/1
  Pref/1 -> Add/1
  Add/1 -> Sum/2
  Step/1 -> Add/2
  Add1/1 -> Sum1/2
  Step1/1 -> Add1/2
  Qref/1 -> Add1/1

== system HVDC_system_original/Control Systems /REC Control/Scaling ==
  Vdc : Inport
  VdVq : Inport  Port=2
  0.8 to 1.2 x Vnom_dc : Saturate  UpperLimit=1.5*Vnom_dc_3L  LowerLimit=0.5*Vnom_dc_3L
  Constant1 : Constant  Value=Vnom_sec_3L
  Gain1 : Gain  Gain=0.5/sqrt(2)*sqrt(3)
  Product : Product  Inputs=*/
  Product1 : Product  Inputs=**
  VdVq* : Outport
  wires:
  Product1/1 -> VdVq*/1
  VdVq/1 -> Product1/1
  Vdc/1 -> 0.8 to 1.2 x Vnom_dc/1
  Product/1 -> Product1/2
  0.8 to 1.2 x Vnom_dc/1 -> Gain1/1
  Gain1/1 -> Product/2
  Constant1/1 -> Product/1

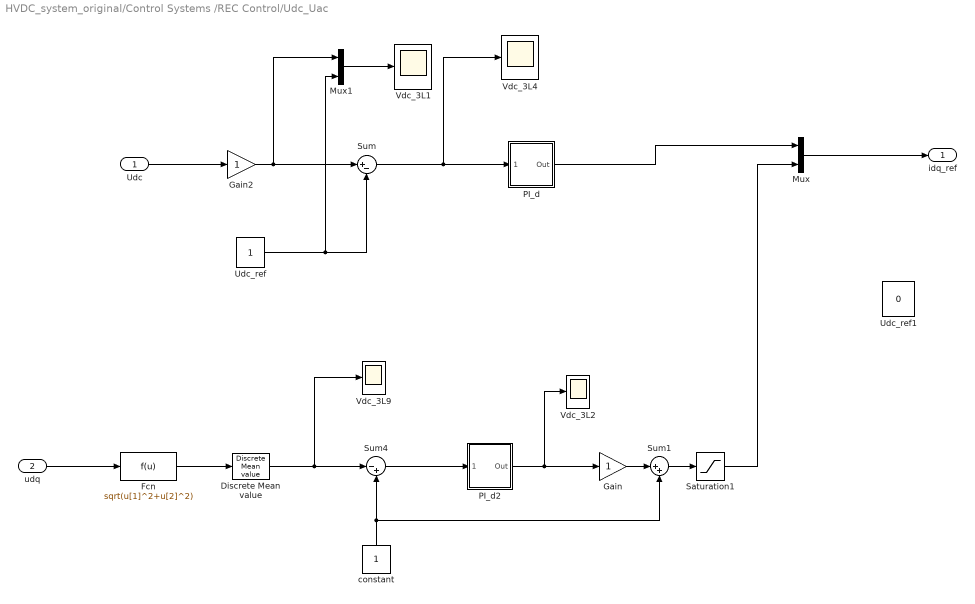
== system HVDC_system_original/Control Systems /REC Control/Udc_Uac ==
  Udc : Inport
  udq : Inport  Port=2
  Discrete Mean value : powerlib_extras/Discrete Measurements/Discrete  Mean value  Freq=60  Vinit=1  Ts=Ts_Control
  Fcn : Fcn  Expr=sqrt(u[1]^2+u[2]^2)  SampleTime=Ts_Control
  Gain : Gain
  Gain2 : Gain
  Mux : Mux  Inputs=2
  Mux1 : Mux  Inputs=2
  PI_d : Subsystem  DialogController=POWERSYS.PowerSysDialog  mask(Discrete PI Controller){Kp=3, Ki=200, Par_Limits=[1.15 -1.15], Init=0, Ts=Ts_Control}
      mask prompts: Kp "Proportional gain (Kp):"; Ki "Integral gain (Ki):"; Par_Limits "Output limits: [ Upper   Lower ]"; Init "Output initial value:"; Ts "Sample time:"
      mask help: This block implements a discrete PI controller.
      mask init:
      | UpperLimit=Par_Limits(1);
      | LowerLimit=Par_Limits(2);
      mask Display: disp('PI');
  PI_d2 : Subsystem  DialogController=POWERSYS.PowerSysDialog  mask(Discrete PI Controller){Kp=0.5, Ki=50, Par_Limits=[0.1 -0.1], Init=0, Ts=Ts_Control}
      mask prompts: Kp "Proportional gain (Kp):"; Ki "Integral gain (Ki):"; Par_Limits "Output limits: [ Upper   Lower ]"; Init "Output initial value:"; Ts "Sample time:"
      mask help: This block implements a discrete PI controller.
      mask init:
      | UpperLimit=Par_Limits(1);
      | LowerLimit=Par_Limits(2);
      mask Display: disp('PI');
  Saturation1 : Saturate  UpperLimit=1.15  LowerLimit=-1.15
  Sum : Sum  Inputs=|+-
  Sum1 : Sum  Inputs=|++
  Sum4 : Sum  Inputs=|-+
  Udc_ref : Constant
  Udc_ref1 : Constant  Value=0
  Vdc_3L{1..2,4,9} (4 alike) : Scope
  constant : Constant  SampleTime=Ts_Control
  idq_ref : Outport
  wires:
  Sum/1 -> Vdc_3L4/1, PI_d/1(Error)
  Mux/1 -> idq_ref/1
  Udc/1 -> Gain2/1
  Saturation1/1 -> Mux/2
  constant/1 -> Sum1/2, Sum4/2
  Sum4/1 -> PI_d2/1(Error)
  PI_d2/1(Out) -> Vdc_3L2/1, Gain/1
  Fcn/1 -> Discrete Mean value/1
  udq/1 -> Fcn/1
  Discrete Mean value/1 -> Vdc_3L9/1, Sum4/1
  Gain/1 -> Sum1/1
  Sum1/1 -> Saturation1/1
  Udc_ref/1 -> Mux1/2, Sum/2
  Gain2/1 -> Mux1/1, Sum/1
  Mux1/1 -> Vdc_3L1/1
  PI_d/1(Out) -> Mux/1

== system HVDC_system_original/Control Systems /SEC Control/PWM Gen 3L ==
  Select : Inport
  Uref : Inport  Port=2
  PWMgen - Averaging : Subsystem
  Pavg_3L : Subsystem
  Switch : Switch  Threshold=1.5  SaturateOnIntegerOverflow=off  InputSameDT=off
  g : Outport
  wires:
  Select/1 -> PWMgen - Averaging/Enable, Switch/2
  PWMgen - Averaging/1(g1_avg) -> Pavg_3L/1(g1)
  Switch/1 -> g/1
  PWMgen - Averaging/2(g4_avg) -> Pavg_3L/2(g4)
  PWMgen - Averaging/3(P) -> Switch/3
  Uref/1 -> PWMgen - Averaging/1(Uref)
  Pavg_3L/1(g) -> Switch/1

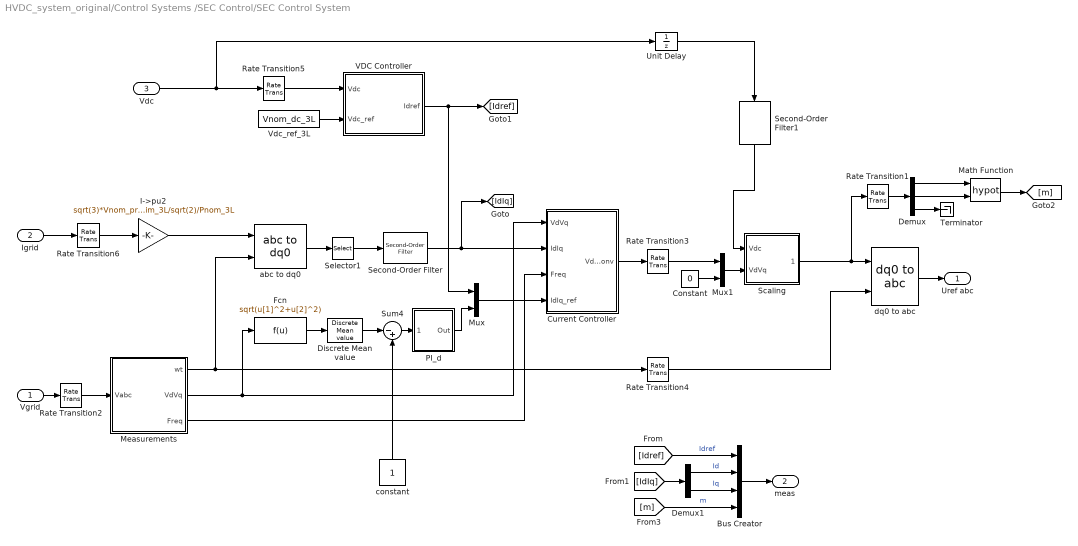
== system HVDC_system_original/Control Systems /SEC Control/SEC Control System ==
  Vgrid : Inport  PortDimensions=3
  Igrid : Inport  Port=2  PortDimensions=3
  Vdc : Inport  Port=3
  Bus Creator : BusCreator  Inputs=4
  Constant : Constant  Value=0
  Current Controller : Subsystem
  Demux : Demux  Outputs=3
  Demux1 : Demux  Outputs=2
  Discrete Mean value : powerlib_extras/Discrete Measurements/Discrete  Mean value  Freq=Fnom  Vinit=1  Ts=Ts_Control
  Fcn : Fcn  Expr=sqrt(u[1]^2+u[2]^2)  SampleTime=Ts_Control
  I->pu2 : Gain  Gain=sqrt(3)*Vnom_prim_3L/sqrt(2)/Pnom_3L  SaturateOnIntegerOverflow=on  OutDataTypeStr=Inherit: Same as input  ParamDataTypeStr=Inherit: Same as input
  Math Function : Math  Operator=hypot  SignedPower=on
  Measurements : Subsystem
  Mux : Mux  Inputs=2
  Mux1 : Mux  Inputs=[2 1]
  PI_d : Subsystem  DialogController=POWERSYS.PowerSysDialog  mask(Discrete PI Controller){Kp=0.5, Ki=50, Par_Limits=[1  -1], Init=0, Ts=Ts_Control}
      mask prompts: Kp "Proportional gain (Kp):"; Ki "Integral gain (Ki):"; Par_Limits "Output limits: [ Upper   Lower ]"; Init "Output initial value:"; Ts "Sample time:"
      mask help: This block implements a discrete PI controller.
      mask init:
      | UpperLimit=Par_Limits(1);
      | LowerLimit=Par_Limits(2);
      mask Display: disp('PI');
  Rate Transition{1..2,5..6} (4 alike) : RateTransition  OutPortSampleTime=Ts_Control
  Rate Transition3 : RateTransition  OutPortSampleTime=Ts_PWM
  Rate Transition4 : RateTransition  OutPortSampleTime=Ts_PWM
  Scaling : Subsystem
  Second-Order Filter : spsSecondOrderFilterLib/Second-Order Filter  FilterType=Lowpass  Fo=Freq_Filter  Zeta=1  Ts=Ts_Control  Initialize=off  Vac_Init="[0,  0,  60]"  Vdc_Init=0  PlotResponse=off  FreqRange=[0, 500, 1]
      settings: LibrarySourceBlock=|
      | sps_lib/Control/Filters/Second-Order
      | Filter
  Second-Order Filter1 : spsSecondOrderFilterLib/Second-Order Filter  FilterType=Lowpass  Fo=Freq_Filter  Zeta=1  Ts=Ts_PWM  Initialize=off  Vac_Init="[0,  0,  60]"  Vdc_Init=0  PlotResponse=off  FreqRange=[0, 500, 1]
      settings: LibrarySourceBlock=|
      | sps_lib/Control/Filters/Second-Order
      | Filter
  Selector1 : Selector  InputPortWidth=3  IndexOptions=Index vector (dialog)  Indices=[1 2]  OutputSizes=1
  Sum4 : Sum  Inputs=|-+
  Terminator : Terminator
  Unit Delay : UnitDelay  SampleTime=Ts_PWM  HasFrameUpgradeWarning=on
  VDC Controller : Subsystem
  Vdc_ref_3L : Constant  Value=Vnom_dc_3L
  abc to dq0 : spsabctodq0Lib/abc to dq0  Alignment=90 degrees behind phase A axis
  constant : Constant  SampleTime=Ts_Control
  dq0 to abc : spsdq0toabcLib/dq0 to abc  Alignment=90 degrees behind phase A axis
  Uref abc : Outport
  meas : Outport  Port=2
  wires:
  Selector1/1 -> Second-Order Filter/1
  I->pu2/1 -> abc to dq0/1
  Igrid/1 -> Rate Transition6/1
  abc to dq0/1 -> Selector1/1
  VDC Controller/1(Idref) -> [Idref], Mux/1
  Scaling/1(VdVq*) -> dq0 to abc/1, Rate Transition1/1
  Mux1/1 -> Scaling/2(VdVq)
  Mux/1 -> Current Controller/4(IdIq_ref)
  Demux/3 -> Terminator/1
  Demux/2 -> Math Function/2
  Demux/1 -> Math Function/1
  Constant/1 -> Mux1/2
  Rate Transition3/1 -> Mux1/1
  Rate Transition4/1 -> dq0 to abc/2
  Current Controller/1(VdVq_conv) -> Rate Transition3/1
  dq0 to abc/1 -> Uref abc/1
  Vgrid/1 -> Rate Transition2/1
  Rate Transition2/1 -> Measurements/1(Vabc)
  Rate Transition6/1 -> I->pu2/1
  Measurements/1(wt) -> Rate Transition4/1, abc to dq0/2
  Measurements/2(VdVq) -> Current Controller/1(VdVq), Fcn/1
  Measurements/3(Freq) -> Current Controller/3(Freq)
  Vdc_ref_3L/1 -> VDC Controller/2(Vdc_ref)
  [Idref] -> Bus Creator/1  "Idref"
  Demux1/1 -> Bus Creator/2  "Id"
  Demux1/2 -> Bus Creator/3  "Iq"
  [m] -> Bus Creator/4  "m"
  [IdIq] -> Demux1/1
  Bus Creator/1 -> meas/1
  Math Function/1 -> [m]
  Rate Transition5/1 -> VDC Controller/1(Vdc)
  Rate Transition1/1 -> Demux/1
  Vdc/1 -> Unit Delay/1, Rate Transition5/1
  Unit Delay/1 -> Second-Order Filter1/1
  Second-Order Filter/1 -> [IdIq], Current Controller/2(IdIq)
  Second-Order Filter1/1 -> Scaling/1(Vdc)
  Fcn/1 -> Discrete Mean value/1
  Discrete Mean value/1 -> Sum4/1
  constant/1 -> Sum4/2
  Sum4/1 -> PI_d/1(Error)
  PI_d/1(Out) -> Mux/2

== system HVDC_system_original/Control Systems /REC Control/Current_control/PI_d ==
  Error : Inport  SampleTime=Ts
  Discrete-Time Integrator : DiscreteIntegrator  InitialCondition=Init  SampleTime=Ts  LimitOutput=on  UpperSaturationLimit=UpperLimit  LowerSaturationLimit=LowerLimit  ICPrevOutput=DiscIntNeverNeededParam  ICPrevScaledInput=DiscIntNeverNeededParam
  Kp4 : Gain  Gain=Kp  SaturateOnIntegerOverflow=on  SampleTime=Ts  OutDataTypeStr=Inherit: Same as input  ParamDataTypeStr=Inherit: Same as input
  Kp5 : Gain  Gain=Ki  SaturateOnIntegerOverflow=on  SampleTime=Ts  OutDataTypeStr=Inherit: Same as input  ParamDataTypeStr=Inherit: Same as input
  Saturation2 : Saturate  UpperLimit=UpperLimit  LowerLimit=LowerLimit  SampleTime=Ts
  Sum6 : Sum  InputSameDT=on  SaturateOnIntegerOverflow=on  SampleTime=Ts  OutDataTypeStr=Inherit: Same as first input
  Zero-Order Hold : ZeroOrderHold  SampleTime=Ts
  Out : Outport  SampleTime=Ts  InitialOutput=0
  wires:
  Saturation2/1 -> Out/1
  Error/1 -> Kp4/1, Kp5/1
  Sum6/1 -> Saturation2/1
  Kp5/1 -> Discrete-Time Integrator/1
  Kp4/1 -> Zero-Order Hold/1
  Discrete-Time Integrator/1 -> Sum6/2
  Zero-Order Hold/1 -> Sum6/1

== system HVDC_system_original/Control Systems /REC Control/Current_control/PI_d1 ==
  Error : Inport  SampleTime=Ts
  Discrete-Time Integrator : DiscreteIntegrator  InitialCondition=Init  SampleTime=Ts  LimitOutput=on  UpperSaturationLimit=UpperLimit  LowerSaturationLimit=LowerLimit  ICPrevOutput=DiscIntNeverNeededParam  ICPrevScaledInput=DiscIntNeverNeededParam
  Kp4 : Gain  Gain=Kp  SaturateOnIntegerOverflow=on  SampleTime=Ts  OutDataTypeStr=Inherit: Same as input  ParamDataTypeStr=Inherit: Same as input
  Kp5 : Gain  Gain=Ki  SaturateOnIntegerOverflow=on  SampleTime=Ts  OutDataTypeStr=Inherit: Same as input  ParamDataTypeStr=Inherit: Same as input
  Saturation2 : Saturate  UpperLimit=UpperLimit  LowerLimit=LowerLimit  SampleTime=Ts
  Sum6 : Sum  InputSameDT=on  SaturateOnIntegerOverflow=on  SampleTime=Ts  OutDataTypeStr=Inherit: Same as first input
  Zero-Order Hold : ZeroOrderHold  SampleTime=Ts
  Out : Outport  SampleTime=Ts  InitialOutput=0
  wires:
  Saturation2/1 -> Out/1
  Error/1 -> Kp4/1, Kp5/1
  Sum6/1 -> Saturation2/1
  Kp5/1 -> Discrete-Time Integrator/1
  Kp4/1 -> Zero-Order Hold/1
  Discrete-Time Integrator/1 -> Sum6/2
  Zero-Order Hold/1 -> Sum6/1

== system HVDC_system_original/Control Systems /REC Control/PLL/PQ ==
  ud : Inport
  id : Inport  Port=2
  uq : Inport  Port=3
  iq : Inport  Port=4
  Add : Sum
  Add1 : Sum  Inputs=+-
  Product{,1..3} (4 alike) : Product
  P : Outport
  Q : Outport  Port=2
  wires:
  id/1 -> Product2/2, Product/2
  Product/1 -> Add/1
  iq/1 -> Product3/1, Product1/2
  uq/1 -> Product2/1, Product1/1
  Product1/1 -> Add/2
  Add/1 -> P/1
  ud/1 -> Product3/2, Product/1
  Product2/1 -> Add1/1
  Product3/1 -> Add1/2
  Add1/1 -> Q/1

== system HVDC_system_original/Control Systems /REC Control/PWM Gen 3L/PWMgen - Averaging ==
  Uref : Inport
  Enable : EnablePort
  Mean : spsMeanLib/Mean  Freq=1/Ts_Power  Vinit=0  Ts=Ts_PWM
  Mean1 : spsMeanLib/Mean  Freq=1/Ts_Power  Vinit=0  Ts=Ts_PWM
  PWM Gen 3L : spsPWMGenerator3LevelLib/PWM Generator (3-Level)  ModulatorType=Three-phase bridge (12 pulses)  ModulatorMode=Unsynchronized  nF=27  Fc=Fc_3L  ModulatingSignals=off  m=0.8  Freq=60  Phase=0  Ts=Ts_PWM
      settings: LibrarySourceBlock=|
      | sps_lib/Power Electronics/Power Electronics Control/PWM Generator
      | (3-Level)
  Selector2 : Selector  InputPortWidth=12  IndexOptions=Index vector (dialog)  Indices="[1  5  9]"  OutputSizes=1
  Selector3 : Selector  InputPortWidth=12  IndexOptions=Index vector (dialog)  Indices="[1  5  9]+3"  OutputSizes=1
  g1_avg : Outport
  g4_avg : Outport  Port=2
  P : Outport  Port=3
  wires:
  Uref/1 -> PWM Gen 3L/1
  PWM Gen 3L/1 -> P/1, Selector2/1, Selector3/1
  Selector3/1 -> Mean1/1  "g4"
  Selector2/1 -> Mean/1  "g1"
  Mean/1 -> g1_avg/1
  Mean1/1 -> g4_avg/1

== system HVDC_system_original/Control Systems /REC Control/PWM Gen 3L/Pavg_3L ==
  g1 : Inport  SampleTime=Ts_PWM
  g4 : Inport  Port=2  SampleTime=Ts_PWM
  Add1 : Sum  Inputs=-+
  Add2 : Sum  Inputs=-+
  Mux2 : Mux  Inputs=[ 3 3 3 3 ]
  Selector1 : Selector  InputPortWidth=12  IndexOptions=Index vector (dialog)  Indices=[1 4 7 10 2 5 8 11 3 6 9 12]  OutputSizes=1
  Zero-Order Hold1 : ZeroOrderHold  SampleTime=Ts_Power
  Zero-Order Hold2 : ZeroOrderHold  SampleTime=Ts_Power
  k1 : Constant
  k3 : Constant
  g : Outport  SampleTime=Ts_Power
  wires:
  Selector1/1 -> g/1
  Mux2/1 -> Selector1/1
  Add1/1 -> Mux2/2  "2abc"
  Add2/1 -> Mux2/3  "3abc"
  Zero-Order Hold2/1 -> Mux2/4, Add1/1  "4abc"
  k1/1 -> Add1/2
  Zero-Order Hold1/1 -> Mux2/1, Add2/1  "1abc"
  k3/1 -> Add2/2
  g1/1 -> Zero-Order Hold1/1
  g4/1 -> Zero-Order Hold2/1

== system HVDC_system_original/Control Systems /REC Control/P_Q/PI_d ==
  Error : Inport  SampleTime=Ts
  Discrete-Time Integrator : DiscreteIntegrator  InitialCondition=Init  SampleTime=Ts  LimitOutput=on  UpperSaturationLimit=UpperLimit  LowerSaturationLimit=LowerLimit  ICPrevOutput=DiscIntNeverNeededParam  ICPrevScaledInput=DiscIntNeverNeededParam
  Kp4 : Gain  Gain=Kp  SaturateOnIntegerOverflow=on  SampleTime=Ts  OutDataTypeStr=Inherit: Same as input  ParamDataTypeStr=Inherit: Same as input
  Kp5 : Gain  Gain=Ki  SaturateOnIntegerOverflow=on  SampleTime=Ts  OutDataTypeStr=Inherit: Same as input  ParamDataTypeStr=Inherit: Same as input
  Saturation2 : Saturate  UpperLimit=UpperLimit  LowerLimit=LowerLimit  SampleTime=Ts
  Sum6 : Sum  InputSameDT=on  SaturateOnIntegerOverflow=on  SampleTime=Ts  OutDataTypeStr=Inherit: Same as first input
  Zero-Order Hold : ZeroOrderHold  SampleTime=Ts
  Out : Outport  SampleTime=Ts  InitialOutput=0
  wires:
  Saturation2/1 -> Out/1
  Error/1 -> Kp4/1, Kp5/1
  Sum6/1 -> Saturation2/1
  Kp5/1 -> Discrete-Time Integrator/1
  Kp4/1 -> Zero-Order Hold/1
  Discrete-Time Integrator/1 -> Sum6/2
  Zero-Order Hold/1 -> Sum6/1

== system HVDC_system_original/Control Systems /REC Control/P_Q/PI_d1 ==
  Error : Inport  SampleTime=Ts
  Discrete-Time Integrator : DiscreteIntegrator  InitialCondition=Init  SampleTime=Ts  LimitOutput=on  UpperSaturationLimit=UpperLimit  LowerSaturationLimit=LowerLimit  ICPrevOutput=DiscIntNeverNeededParam  ICPrevScaledInput=DiscIntNeverNeededParam
  Kp4 : Gain  Gain=Kp  SaturateOnIntegerOverflow=on  SampleTime=Ts  OutDataTypeStr=Inherit: Same as input  ParamDataTypeStr=Inherit: Same as input
  Kp5 : Gain  Gain=Ki  SaturateOnIntegerOverflow=on  SampleTime=Ts  OutDataTypeStr=Inherit: Same as input  ParamDataTypeStr=Inherit: Same as input
  Saturation2 : Saturate  UpperLimit=UpperLimit  LowerLimit=LowerLimit  SampleTime=Ts
  Sum6 : Sum  InputSameDT=on  SaturateOnIntegerOverflow=on  SampleTime=Ts  OutDataTypeStr=Inherit: Same as first input
  Zero-Order Hold : ZeroOrderHold  SampleTime=Ts
  Out : Outport  SampleTime=Ts  InitialOutput=0
  wires:
  Saturation2/1 -> Out/1
  Error/1 -> Kp4/1, Kp5/1
  Sum6/1 -> Saturation2/1
  Kp5/1 -> Discrete-Time Integrator/1
  Kp4/1 -> Zero-Order Hold/1
  Discrete-Time Integrator/1 -> Sum6/2
  Zero-Order Hold/1 -> Sum6/1

== system HVDC_system_original/Control Systems /REC Control/Udc_Uac/PI_d ==
  Error : Inport  SampleTime=Ts
  Discrete-Time Integrator : DiscreteIntegrator  InitialCondition=Init  SampleTime=Ts  LimitOutput=on  UpperSaturationLimit=UpperLimit  LowerSaturationLimit=LowerLimit  ICPrevOutput=DiscIntNeverNeededParam  ICPrevScaledInput=DiscIntNeverNeededParam
  Kp4 : Gain  Gain=Kp  SaturateOnIntegerOverflow=on  SampleTime=Ts  OutDataTypeStr=Inherit: Same as input  ParamDataTypeStr=Inherit: Same as input
  Kp5 : Gain  Gain=Ki  SaturateOnIntegerOverflow=on  SampleTime=Ts  OutDataTypeStr=Inherit: Same as input  ParamDataTypeStr=Inherit: Same as input
  Saturation2 : Saturate  UpperLimit=UpperLimit  LowerLimit=LowerLimit  SampleTime=Ts
  Sum6 : Sum  InputSameDT=on  SaturateOnIntegerOverflow=on  SampleTime=Ts  OutDataTypeStr=Inherit: Same as first input
  Zero-Order Hold : ZeroOrderHold  SampleTime=Ts
  Out : Outport  SampleTime=Ts  InitialOutput=0
  wires:
  Saturation2/1 -> Out/1
  Error/1 -> Kp4/1, Kp5/1
  Sum6/1 -> Saturation2/1
  Kp5/1 -> Discrete-Time Integrator/1
  Kp4/1 -> Zero-Order Hold/1
  Discrete-Time Integrator/1 -> Sum6/2
  Zero-Order Hold/1 -> Sum6/1
